simulink model "px4demo_rgbled"  (R2016a)
settings: Solver=FixedStepDiscrete  SolverMode=SingleTasking  StartTime=0.0  StopTime=10.0  RelTol=1e-3
PostLoadFcn:
  | Ts = 1/250;
undefined symbols (not defined in the file or in its folder): RGBLED_COLOR_ENUM, RGBLED_MODE_ENUM
libraries: pixhawk_slib_sensors_actuators x1
settings Model: Creator=skuznick  LastModifiedBy=darenlee
settings DataIOCC: LimitDataPoints=on  SaveFormat=Array
settings OptimizationCC: DefaultParameterBehavior=Inlined  OptimizeModelRefInitCode=on  LifeSpan=1  MaxStackSize=64
settings DebuggingCC: SolverPrmCheckMsg=warning  AllowSymbolicDim=off
settings HardwareCC: ProdBitPerPointer=32  ProdLargestAtomicInteger=Long  ProdLargestAtomicFloat=Double  ProdWordSize=32  ProdHWDeviceType=ARM Compatible->ARM Cortex
settings ModelReferenceCC: PropagateSignalLabelsOutOfModel=off
settings RTWCC: SystemTargetFile=ert.tlc  HardwareBoard=Pixhawk PX4  TemplateMakefile=ert_default_tmf  GenerateReport=on  Toolchain=Pixhawk Toolchain  IncludeHyperlinkInReport=on  LaunchReport=on  GenerateTraceReport=on  GenerateCodeMetricsReport=on
settings CodeAppCC: IgnoreCustomStorageClasses=off
settings ERTTargetCC: ERTCustomFileTemplate=PX4_codertarget_file_process.tlc  ConvertIfToSwitch=off  SuppressUnreachableDefaultCases=off
settings ConfigComp: CovModelRefEnable=Off  CovSFcnEnable=off

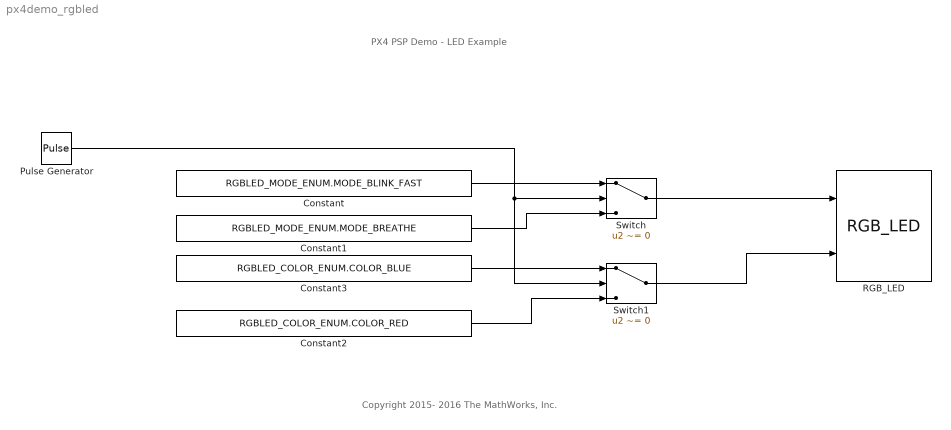
== system px4demo_rgbled ==
  note: PX4 PSP Demo - LED Example
  note: Copyright 2015- 2016 The MathWorks, Inc.
  Constant : Constant  Value=RGBLED_MODE_ENUM.MODE_BLINK_FAST  OutDataTypeStr=Enum: RGBLED_MODE_ENUM
  Constant1 : Constant  Value=RGBLED_MODE_ENUM.MODE_BREATHE  OutDataTypeStr=Enum: RGBLED_MODE_ENUM
  Constant2 : Constant  Value=RGBLED_COLOR_ENUM.COLOR_RED  OutDataTypeStr=Enum: RGBLED_COLOR_ENUM
  Constant3 : Constant  Value=RGBLED_COLOR_ENUM.COLOR_BLUE  OutDataTypeStr=Enum: RGBLED_COLOR_ENUM
  Pulse Generator : DiscretePulseGenerator  PulseType=Time based  PulseWidth=50
  RGB_LED : pixhawk_slib_sensors_actuators/RGB_LED
  Switch : Switch  Criteria=u2 ~= 0  Threshold=1500
  Switch1 : Switch  Criteria=u2 ~= 0  Threshold=1500
  wires:
  Switch/1 -> RGB_LED/1
  Switch1/1 -> RGB_LED/2
  Constant/1 -> Switch/1
  Constant1/1 -> Switch/3
  Constant3/1 -> Switch1/1
  Constant2/1 -> Switch1/3
  Pulse Generator/1 -> Switch1/2, Switch/2
